simulink model "FuzzyPID_PMSM"  (R2022a)
settings: Solver=VariableStepAuto  StartTime=0.0  StopTime=20  RelTol=1e-3
settings Model: Creator=abang  LastModifiedBy=ASUS
settings DebuggingCC: UnconnectedInputMsg=warning  UnconnectedOutputMsg=warning  UnconnectedLineMsg=warning
settings RTWCC: DLArmComputeVersion=19.05

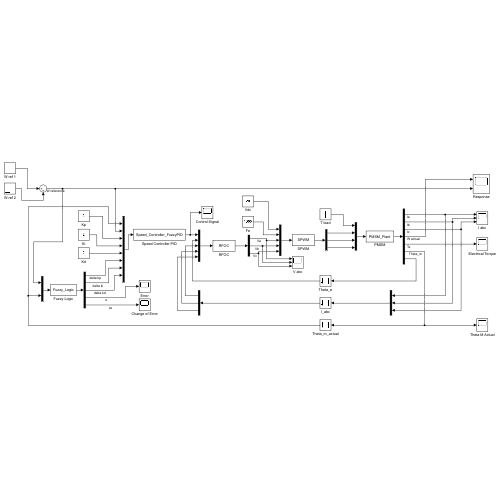
[thumbnail: Simulink's stored preview of the top-level diagram]
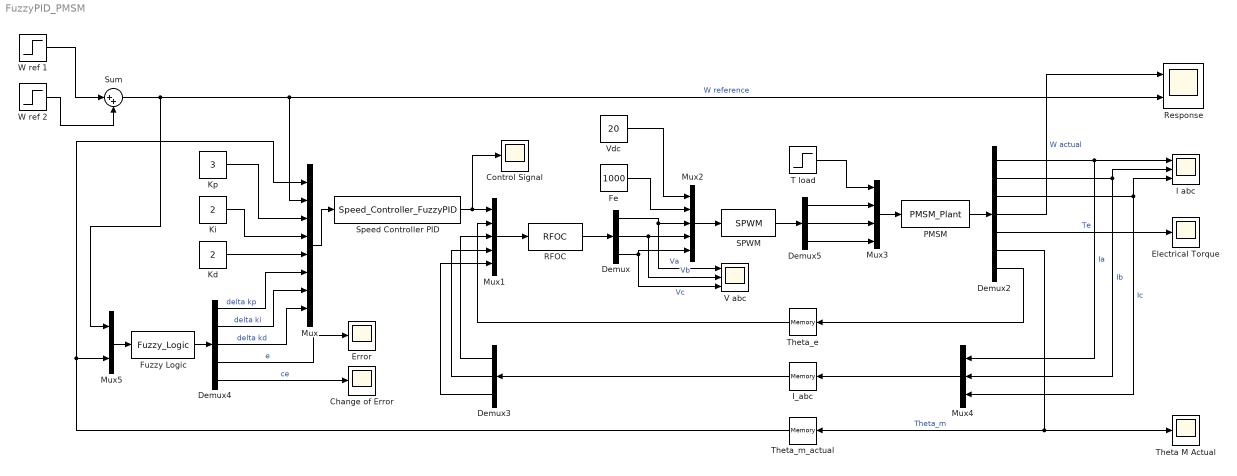
== system FuzzyPID_PMSM ==
  Change of Error : Scope
  Control Signal : Scope
  Demux : Demux  Outputs=3
  Demux2 : Demux  Outputs=7
  Demux3 : Demux  Outputs=3
  Demux4 : Demux  Outputs=5
  Demux5 : Demux  Outputs=3
  Electrical Torque : Scope
  Error : Scope
  Fe : Constant  Value=1000
  Fuzzy Logic : S-Function  FunctionName=Fuzzy_Logic  SFunctionDeploymentMode=off  EnableBusSupport=off
  I abc : Scope  NumInputPorts=3
  I_abc : Memory
  Kd : Constant  Value=2
  Ki : Constant  Value=2
  Kp : Constant  Value=3
  Mux : Mux  Inputs=8
  Mux1 : Mux  Inputs=5
  Mux2 : Mux  Inputs=5
  Mux3 : Mux
  Mux4 : Mux  Inputs=3
  Mux5 : Mux  Inputs=2
  PMSM : S-Function  FunctionName=PMSM_Plant  SFunctionDeploymentMode=off  EnableBusSupport=off
  RFOC : S-Function  FunctionName=RFOC  SFunctionDeploymentMode=off  EnableBusSupport=off
  Response : Scope  NumInputPorts=2
  SPWM : S-Function  FunctionName=SPWM  SFunctionDeploymentMode=off  EnableBusSupport=off
  Speed Controller PID : S-Function  FunctionName=Speed_Controller_FuzzyPID  SFunctionDeploymentMode=off  EnableBusSupport=off
  Sum : Sum  Inputs=|++
  T load : Step  Time=10  After=0  SampleTime=0
  Theta M Actual : Scope
  Theta_e : Memory
  Theta_m_actual : Memory
  V abc : Scope  NumInputPorts=3
  Vdc : Constant  Value=20
  W ref 1 : Step  Time=3  Before=5  After=10  SampleTime=0
  W ref 2 : Step  Time=6  After=5  SampleTime=0
  wires:
  Mux/1 -> Speed Controller PID/1
  Mux2/1 -> SPWM/1
  Demux/1 -> Mux2/3, V abc/1  "Va"
  Demux/2 -> Mux2/4, V abc/2  "Vb"
  Demux/3 -> Mux2/5, V abc/3  "Vc"
  Mux3/1 -> PMSM/1
  PMSM/1 -> Demux2/1
  Demux2/1 -> Mux4/1, I abc/1  "Ia"
  Demux2/6 -> Theta_m_actual/1, Theta M Actual/1  "Theta_m"
  RFOC/1 -> Demux/1
  Mux1/1 -> RFOC/1
  Speed Controller PID/1 -> Control Signal/1, Mux1/1
  Vdc/1 -> Mux2/1
  Fe/1 -> Mux2/2
  T load/1 -> Mux3/1
  Demux2/2 -> Mux4/2, I abc/2  "Ib"
  Demux2/3 -> Mux4/3, I abc/3  "Ic"
  Demux2/4 -> Response/1  "W actual"
  Demux2/5 -> Electrical Torque/1  "Te"
  Demux2/7 -> Theta_e/1
  Theta_e/1 -> Mux1/2
  Demux3/1 -> Mux1/3
  Demux3/2 -> Mux1/4
  Demux3/3 -> Mux1/5
  Mux4/1 -> I_abc/1
  I_abc/1 -> Demux3/1
  Sum/1 -> Mux/2, Response/2, Mux5/1  "W reference"
  Theta_m_actual/1 -> Mux/1, Mux5/2
  Kp/1 -> Mux/3
  Ki/1 -> Mux/4
  Kd/1 -> Mux/5
  Mux5/1 -> Fuzzy Logic/1
  Fuzzy Logic/1 -> Demux4/1
  Demux4/1 -> Mux/6  "delta kp"
  Demux4/2 -> Mux/7  "delta ki"
  Demux4/3 -> Mux/8  "delta kd"
  Demux4/4 -> Error/1  "e"
  Demux4/5 -> Change of Error/1  "ce"
  SPWM/1 -> Demux5/1
  Demux5/3 -> Mux3/4
  Demux5/2 -> Mux3/3
  Demux5/1 -> Mux3/2
  W ref 1/1 -> Sum/1
  W ref 2/1 -> Sum/2
